simulink model "pitch_loop"  (R2016a)
settings: Solver=VariableStepAuto  StartTime=0.0  StopTime=50  RelTol=1e-3
values from neighbouring files (symbols this model uses):
  a_theta1 = 0.6984    [tune_pitch.m]
  a_theta2 = 27.1682    [tune_pitch.m]
  a_theta3 = -35.7476    [tune_pitch.m]
  pitch_kd = (2 * zeta_pitch * wn_pitch - a_theta1) / a_theta3    [tune_pitch.m]
  pitch_kp = (wn_pitch^2 - a_theta2) / a_theta3    [tune_pitch.m]
settings Model: Creator=andreanv  LastModifiedBy=andreanv

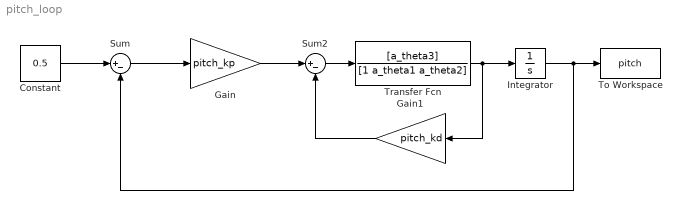
== system pitch_loop ==
  Constant : Constant  Value=0.5
  Gain : Gain  Gain=pitch_kp
  Gain1 : Gain  Gain=pitch_kd
  Integrator : Integrator
  Sum : Sum  Inputs=|+-
  Sum2 : Sum  Inputs=|+-
  To Workspace : ToWorkspace  VariableName=pitch  SaveFormat=Timeseries  SampleTime=-1
  Transfer Fcn : TransferFcn  Numerator=[a_theta3]  Denominator=[1 a_theta1 a_theta2]
  wires:
  Constant/1 -> Sum/1
  Sum/1 -> Gain/1
  Sum2/1 -> Transfer Fcn/1
  Transfer Fcn/1 -> Gain1/1, Integrator/1
  Integrator/1 -> Sum/2, To Workspace/1
  Gain/1 -> Sum2/1
  Gain1/1 -> Sum2/2
